simulink model "idealmodel1"  (Simulink 7.5)
settings: Solver=ode45  StartTime=0.0  StopTime=5.0  RelTol=1e-3
libraries: powerlib x3
settings Model: Creator=comp  LastModifiedBy=comp

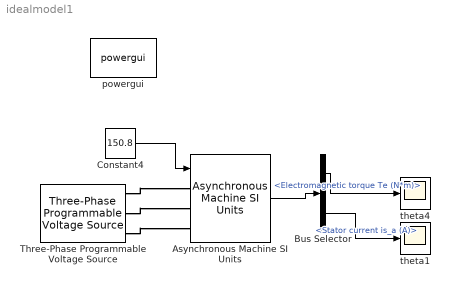
== system idealmodel1 ==
  Asynchronous Machine SI Units : powerlib/Machines/Asynchronous Machine SI Units  DialogController=POWERSYS.PowerSysDialog  SystemSampleTime=-1  PresetModel=No  MechanicalLoad=Speed w  ShowDetailedParameters=on  RotorType=Squirrel-cage  ReferenceFrame=Stationary  NominalParameters=[149.2e3 400 50]  Stator=[14.85e-3 .3027e-3]  Rotor=[9.295e-3 .3027e-3]  Lm=10.46e-3  Mechanical=[0.0131 0.002985 2]  PolePairs=2  InitialConditions=[1 0 0 0 0 0 0 0]  Units=SI  LoadFlowParameters=1492000  SimulateSaturation=off  Saturation=[14.03593122, 27.81365428, 53.79336849, 72.68890987, 97.98006896, 148.6815601, 215.7428561, 302.9841135, 428.7778367 ; 230, 322, 414, 460, 506, 552, 598, 644, 690]  TsPowergui=0  TsBlock=-1  IterativeModel=Forward Euler
  Bus Selector : BusSelector  OutputSignals=Mechanical.Electromagnetic torque Te (N*m),Stator measurements.Stator current is_a (A)
  Constant4 : Constant  Value=150.8  OutDataType=fixdt(1, 16)  OutScaling=2^0
  Three-Phase Programmable Voltage Source : powerlib/Electrical Sources/Three-Phase Programmable Voltage Source  DialogController=POWERSYS.PowerSysDialog  SystemSampleTime=-1  PositiveSequence="[316  0 50]"  VariationEntity=None  VariationType=Step  VariationStep=0.5  VariationRate=10  VariationMagnitude=0.3  VariationFrequency=2  VariationTiming=[1 2]  VariationPhaseA=off  Amplitudes=[1 0.8 1.2 1.0]  TimeValues=[0 0.1 0.15 0.2]  HarmonicGeneration=off  HarmonicA=[3 0.2 -25 0]  HarmonicB=[2 0.15 35 2]  Timing="[0.05  3]"
  powergui : powerlib/powergui  Priority=1  SystemSampleTime=-1  SimulationMode=Discrete  SampleTime=50e-6  frequency=60  SPID=off  DisableSnubberDevices=off  DisableRonSwitches=off  DisableVfSwitches=off  SwTol=0  Interpol=off  frequencyindice=50  echomessages=off  HookPort=off  DisplayEquations=off  FunctionMessages=off  EnableUseOfTLC=off  x0status=blocks  RestoreLinks=warning  ResistiveCurrentMeasurement=off  Ylog=off  Xlog=on  ShowGrid=off  save=off  variable=ZData  ZoomFFT=off  StartTime=0.0  cycles=1  DisplayStyle=1  FreqAxis=off  MaxFrequency=1000  frequencyindicesteady=1  display=off  methode=off
  theta1 : Scope
      settings: TimeRange=5  YMin=-1200  YMax=1200
  theta4 : Scope
      settings: TimeRange=5  YMin=1741.65  YMax=1741.65
  wires:
  Constant4/1 -> Asynchronous Machine SI Units/1
  Asynchronous Machine SI Units/1 -> Bus Selector/1
  Bus Selector/1 -> theta4/1  "<Electromagnetic torque Te (N*m)>"
  Bus Selector/2 -> theta1/1  "<Stator current is_a (A)>"
  connections:
  Three-Phase Programmable Voltage Source/RConn3 -- Asynchronous Machine SI Units/LConn3
  Three-Phase Programmable Voltage Source/RConn2 -- Asynchronous Machine SI Units/LConn2
  Three-Phase Programmable Voltage Source/RConn1 -- Asynchronous Machine SI Units/LConn1
